simulink model "Neuron_Final"  (R2018a)
settings: Solver=VariableStepAuto  StartTime=0.0  StopTime=7200  RelTol=1e-3
settings Model: Creator=andys  LastModifiedBy=andys
settings CodeAppCC: StateflowObjectComments=on

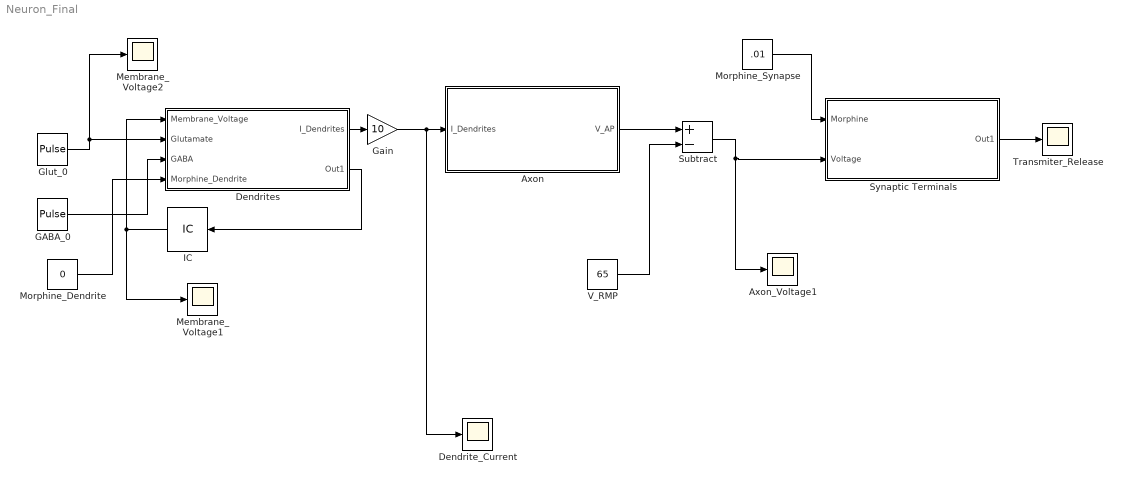
== system Neuron_Final ==
  Axon : Subsystem
  Axon_Voltage1 : Scope
  Dendrite_Current : Scope
  Dendrites : Subsystem
  GABA_0 : DiscretePulseGenerator  PulseType=Time based  Amplitude=0  Period=500  PulseWidth=0.1  PhaseDelay=500
  Gain : Gain  Gain=10
  Glut_0 : DiscretePulseGenerator  PulseType=Time based  Period=500  PulseWidth=0.1  PhaseDelay=500
  IC : InitialCondition  Value=-65
  Membrane_Voltage1 : Scope
  Membrane_Voltage2 : Scope
  Morphine_Dendrite : Constant  Value=0
  Morphine_Synapse : Constant  Value=.01
  Subtract : Sum  Inputs=+-
  Synaptic Terminals : Subsystem
  Transmiter_Release : Scope
  V_RMP : Constant  Value=65
  wires:
  Synaptic Terminals/1(Out1) -> Transmiter_Release/1
  Dendrites/1(I_Dendrites) -> Gain/1
  Glut_0/1 -> Dendrites/2(Glutamate), Membrane_Voltage2/1
  Dendrites/2(Out1) -> IC/1
  V_RMP/1 -> Subtract/2
  Subtract/1 -> Synaptic Terminals/2(Voltage), Axon_Voltage1/1
  IC/1 -> Dendrites/1(Membrane_Voltage), Membrane_Voltage1/1
  Axon/1(V_AP) -> Subtract/1
  Gain/1 -> Axon/1(I_Dendrites), Dendrite_Current/1
  Morphine_Dendrite/1 -> Dendrites/4(Morphine_Dendrite)
  Morphine_Synapse/1 -> Synaptic Terminals/1(Morphine)
  GABA_0/1 -> Dendrites/3(GABA)

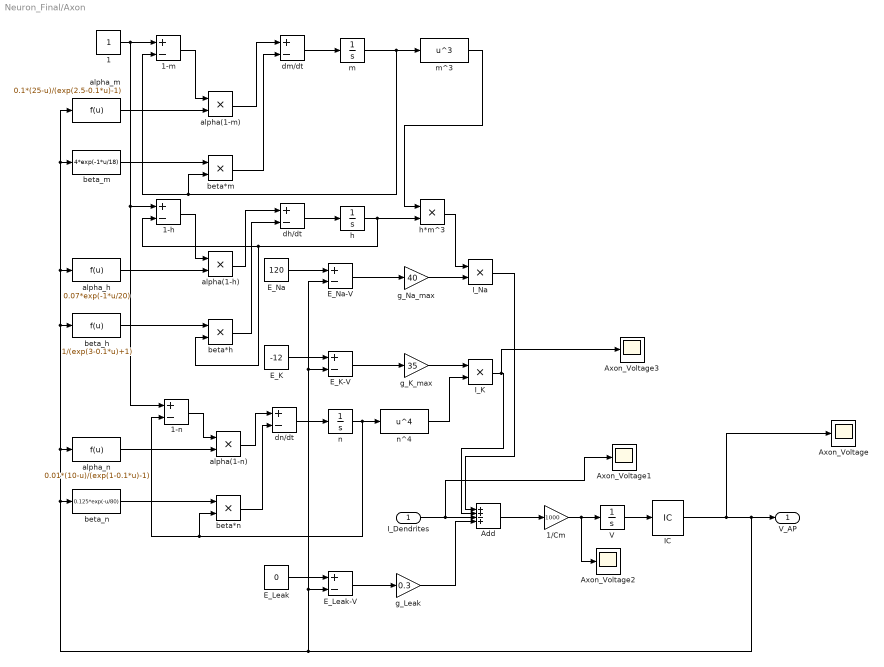
== system Neuron_Final/Axon ==
  I_Dendrites : Inport
  1 : Constant
  1-h : Sum  Inputs=+-
  1-m : Sum  Inputs=+-
  1-n : Sum  Inputs=+-
  1/Cm : Gain  Gain=1000
  Add : Sum  Inputs=++-+
  Axon_Voltage{,1..3} (4 alike) : Scope
  E_K : Constant  Value=-12
  E_K-V : Sum  Inputs=+-
  E_Leak : Constant  Value=0
  E_Leak-V : Sum  Inputs=+-
  E_Na : Constant  Value=120
  E_Na-V : Sum  Inputs=+-
  IC : InitialCondition  Value=0
  I_K : Product
  I_Na : Product
  V : Integrator
  alpha(1-h) : Product
  alpha(1-m) : Product
  alpha(1-n) : Product
  alpha_h : Fcn  Expr=0.07*exp(-1*u/20)
  alpha_m : Fcn  Expr=0.1*(25-u)/(exp(2.5-0.1*u)-1)
  alpha_n : Fcn  Expr=0.01*(10-u)/(exp(1-0.1*u)-1)
  beta*h : Product
  beta*m : Product
  beta*n : Product
  beta_h : Fcn  Expr=1/(exp(3-0.1*u)+1)
  beta_m : Fcn  Expr=4*exp(-1*u/18)
  beta_n : Fcn  Expr=0.125*exp(-u/80)
  dh/dt : Sum  Inputs=+-
  dm/dt : Sum  Inputs=+-
  dn/dt : Sum  Inputs=+-
  g_K_max : Gain  Gain=35
  g_Leak : Gain  Gain=0.3
  g_Na_max : Gain  Gain=40
  h : Integrator
  h*m^3 : Product
  m : Integrator
  m^3 : Fcn  Expr=u^3
  n : Integrator
  n^4 : Fcn  Expr=u^4
  V_AP : Outport
  wires:
  V/1 -> IC/1
  1/Cm/1 -> Axon_Voltage2/1, V/1
  E_Na/1 -> E_Na-V/1
  E_K/1 -> E_K-V/1
  E_Leak/1 -> E_Leak-V/1
  E_Leak-V/1 -> g_Leak/1
  E_K-V/1 -> g_K_max/1
  E_Na-V/1 -> g_Na_max/1
  Add/1 -> 1/Cm/1
  g_Leak/1 -> Add/4
  I_Dendrites/1 -> Axon_Voltage1/1, Add/3
  g_Na_max/1 -> I_Na/2
  g_K_max/1 -> I_K/1
  I_K/1 -> Axon_Voltage3/1, Add/2
  I_Na/1 -> Add/1
  IC/1 -> Axon_Voltage/1, alpha_m/1, beta_m/1, alpha_h/1, beta_h/1, alpha_n/1, beta_n/1, E_Na-V/2, E_K-V/2, E_Leak-V/2, V_AP/1
  n^4/1 -> I_K/2
  h*m^3/1 -> I_Na/1
  n/1 -> beta*n/2, 1-n/2, n^4/1
  m/1 -> m^3/1, beta*m/2, 1-m/2
  m^3/1 -> h*m^3/1
  h/1 -> 1-h/2, beta*h/2, h*m^3/2
  dn/dt/1 -> n/1
  dm/dt/1 -> m/1
  dh/dt/1 -> h/1
  1/1 -> 1-m/1, 1-h/1, 1-n/1
  alpha_m/1 -> alpha(1-m)/2
  1-m/1 -> alpha(1-m)/1
  alpha(1-m)/1 -> dm/dt/1
  beta_m/1 -> beta*m/1
  beta*m/1 -> dm/dt/2
  beta_h/1 -> beta*h/1
  alpha_h/1 -> alpha(1-h)/2
  1-h/1 -> alpha(1-h)/1
  alpha(1-h)/1 -> dh/dt/1
  beta*h/1 -> dh/dt/2
  1-n/1 -> alpha(1-n)/1
  alpha_n/1 -> alpha(1-n)/2
  alpha(1-n)/1 -> dn/dt/1
  beta_n/1 -> beta*n/1
  beta*n/1 -> dn/dt/2

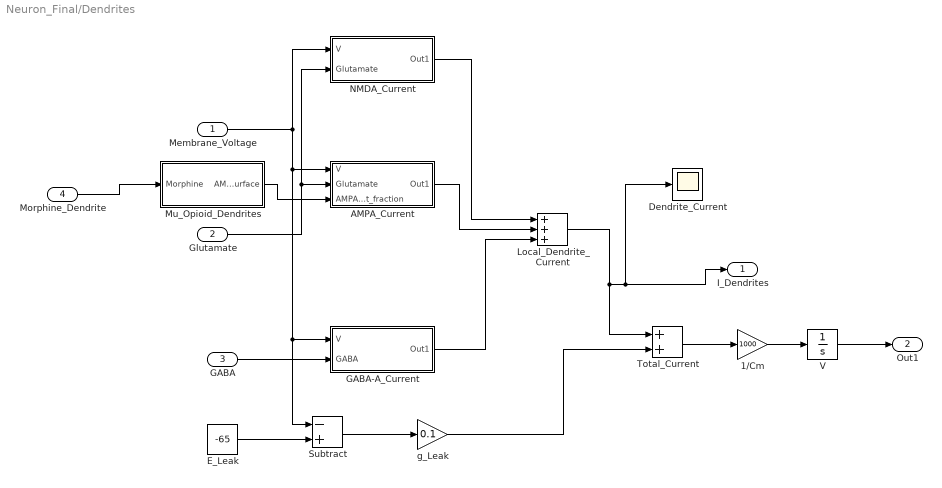
== system Neuron_Final/Dendrites ==
  Membrane_Voltage : Inport
  Glutamate : Inport  Port=2
  GABA : Inport  Port=3
  Morphine_Dendrite : Inport  Port=4
  1/Cm : Gain  Gain=1000
  AMPA_Current : Subsystem
  Dendrite_Current : Scope
  E_Leak : Constant  Value=-65
  GABA-A_Current : Subsystem
  Local_Dendrite_Current : Sum  Inputs=+++
  Mu_Opioid_Dendrites : Subsystem
  NMDA_Current : Subsystem
  Subtract : Sum  Inputs=-+
  Total_Current : Sum
  V : Integrator
  g_Leak : Gain  Gain=0.1
  I_Dendrites : Outport
  Out1 : Outport  Port=2
  wires:
  Membrane_Voltage/1 -> NMDA_Current/1(V), Subtract/1, GABA-A_Current/1(V), AMPA_Current/1(V)
  Glutamate/1 -> NMDA_Current/2(Glutamate), AMPA_Current/2(Glutamate)
  GABA/1 -> GABA-A_Current/2(GABA)
  AMPA_Current/1(Out1) -> Local_Dendrite_Current/2
  GABA-A_Current/1(Out1) -> Local_Dendrite_Current/3
  Local_Dendrite_Current/1 -> Dendrite_Current/1, I_Dendrites/1, Total_Current/1
  Total_Current/1 -> 1/Cm/1
  1/Cm/1 -> V/1
  V/1 -> Out1/1
  E_Leak/1 -> Subtract/2
  Subtract/1 -> g_Leak/1
  g_Leak/1 -> Total_Current/2
  NMDA_Current/1(Out1) -> Local_Dendrite_Current/1
  Morphine_Dendrite/1 -> Mu_Opioid_Dendrites/1("Morphine ")
  Mu_Opioid_Dendrites/1(AMPA_Surface) -> AMPA_Current/3(AMPA_current_fraction)

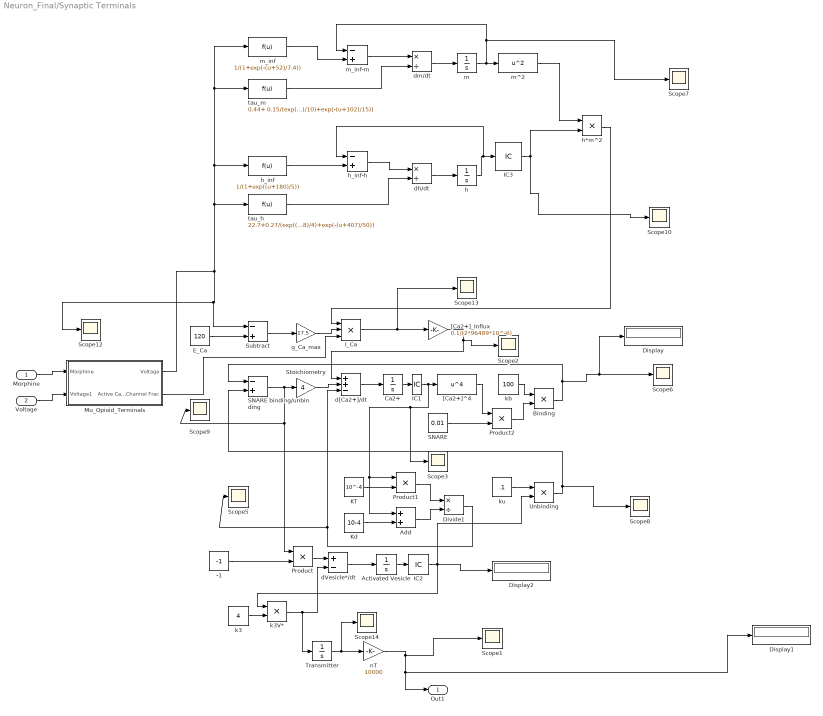
== system Neuron_Final/Synaptic Terminals ==
  Morphine : Inport
  Voltage : Inport  Port=2
  -1 : Constant  Value=-1
  Activated Vesicle : Integrator
  Add : Sum
  Binding : Product
  Ca2+ : Integrator
  Display : Display
  Display1 : Display
  Display2 : Display
  Divide1 : Product  Inputs=*/
  E_Ca : Constant  Value=120
  IC1 : InitialCondition  Value=0
  IC2 : InitialCondition  Value=0
  IC3 : InitialCondition
  I_Ca : Product  Inputs=3
  KT : Constant  Value=10^-4
  Kd : Constant  Value=10-4
  Mu_Opioid_Terminals : Subsystem
  Product : Product
  Product1 : Product
  Product2 : Product
  SNARE : Constant  Value=0.01
  SNARE binding/unbinding : Sum  Inputs=-+
  Scope{1..3,5..10,12..14} (12 alike) : Scope
  Stoichiometry : Gain  Gain=4
  Subtract : Sum  Inputs=-+
  Transmitter : Integrator
  Unbinding : Product
  "[Ca2+]^4" : Fcn  Expr=u^4
  "[Ca2+]_Influx" : Gain  Gain=0.1/(2*96489*10^-6)
  dVesicle*/dt : Sum  Inputs=+-
  d[Ca2+]/dt : Sum  Inputs=++-
  dh/dt : Product  Inputs=*/
  dm/dt : Product  Inputs=*/
  g_Ca_max : Gain  Gain=17.5
  h : Integrator
  h*m^2 : Product
  h_inf : Fcn  Expr=1/(1+exp((u+180)/5))
  h_inf-h : Sum  Inputs=-+
  k3 : Constant  Value=4
  k3V* : Product
  kb : Constant  Value=100
  ku : Constant  Value=.1
  m : Integrator
  m^2 : Fcn  Expr=u^2
  m_inf : Fcn  Expr=1/(1+exp(-(u+52)/7.4))
  m_inf-m : Sum  Inputs=-+
  nT : Gain  Gain=10000
  tau_h : Fcn  Expr=22.7+0.27/(exp((u+48)/4)+exp(-(u+407)/50))
  tau_m : Fcn  Expr=0.44+ 0.15/(exp((u+27)/10)+exp(-(u+102)/15))
  Out1 : Outport
  wires:
  d[Ca2+]/dt/1 -> Ca2+/1
  dVesicle*/dt/1 -> Activated Vesicle/1
  k3V*/1 -> Transmitter/1, dVesicle*/dt/2
  k3/1 -> k3V*/2
  Activated Vesicle/1 -> IC2/1
  Transmitter/1 -> Scope14/1, nT/1
  nT/1 -> Scope1/1, Display1/1, Out1/1
  kb/1 -> Binding/1
  E_Ca/1 -> Subtract/2
  Subtract/1 -> g_Ca_max/1
  g_Ca_max/1 -> I_Ca/2
  m/1 -> m_inf-m/1, Scope7/1, m^2/1
  m^2/1 -> h*m^2/1
  h*m^2/1 -> I_Ca/1
  I_Ca/1 -> Scope13/1, "[Ca2+]_Influx"/1
  "[Ca2+]_Influx"/1 -> Scope2/1, d[Ca2+]/dt/1
  SNARE binding/unbinding/1 -> Stoichiometry/1, Scope9/1, Product/1
  Stoichiometry/1 -> d[Ca2+]/dt/2
  Binding/1 -> Display/1, Scope6/1, SNARE binding/unbinding/1
  Unbinding/1 -> Scope8/1, SNARE binding/unbinding/2
  Ca2+/1 -> IC1/1
  IC1/1 -> Scope3/1, Add/1, Product1/1, "[Ca2+]^4"/1
  ku/1 -> Unbinding/1
  IC2/1 -> Display2/1, k3V*/1, Unbinding/2
  -1/1 -> Product/2
  Product/1 -> dVesicle*/dt/1
  Kd/1 -> Add/2
  KT/1 -> Product1/2
  Product1/1 -> Divide1/1
  Add/1 -> Divide1/2
  Divide1/1 -> Scope5/1, d[Ca2+]/dt/3
  h/1 -> h_inf-h/1, IC3/1
  m_inf/1 -> m_inf-m/2
  m_inf-m/1 -> dm/dt/1
  tau_m/1 -> dm/dt/2
  dm/dt/1 -> m/1
  dh/dt/1 -> h/1
  h_inf/1 -> h_inf-h/2
  h_inf-h/1 -> dh/dt/1
  tau_h/1 -> dh/dt/2
  IC3/1 -> Scope10/1, h*m^2/2
  "[Ca2+]^4"/1 -> Product2/1
  Product2/1 -> Binding/2
  SNARE/1 -> Product2/2
  Mu_Opioid_Terminals/1(Voltage) -> h_inf/1, tau_m/1, m_inf/1, tau_h/1, Subtract/1, Scope12/1
  Morphine/1 -> Mu_Opioid_Terminals/1(Morphine)
  Mu_Opioid_Terminals/2(Active Ca Channel Frac) -> I_Ca/3
  Voltage/1 -> Mu_Opioid_Terminals/2(Voltage1)

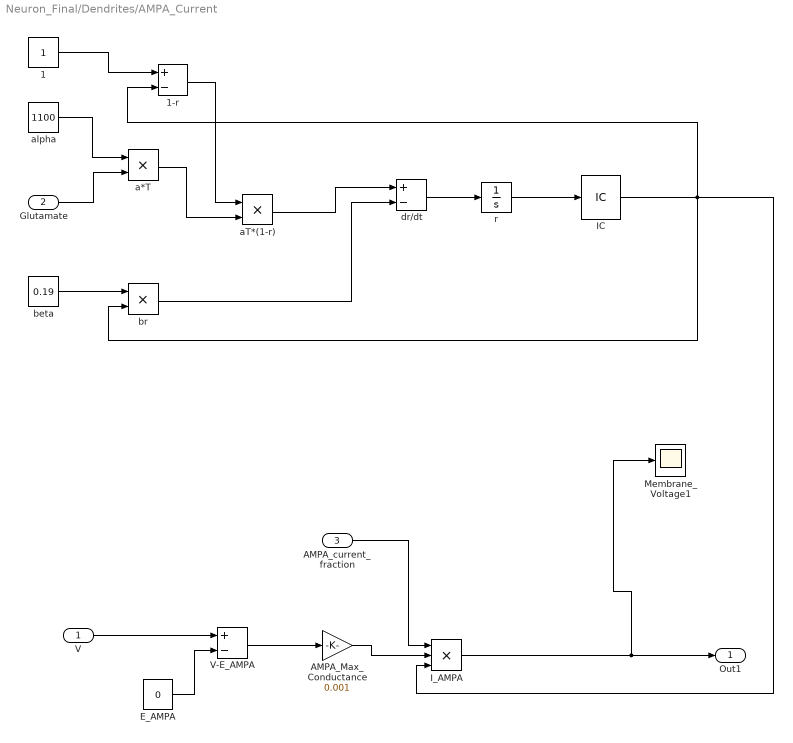
== system Neuron_Final/Dendrites/AMPA_Current ==
  V : Inport
  Glutamate : Inport  Port=2
  AMPA_current_fraction : Inport  Port=3
  1 : Constant
  1-r : Sum  Inputs=+-
  AMPA_Max_Conductance : Gain  Gain=0.001
  E_AMPA : Constant  Value=0
  IC : InitialCondition  Value=0
  I_AMPA : Product  Inputs=3
  Membrane_Voltage1 : Scope
  V-E_AMPA : Sum  Inputs=+-
  a*T : Product
  aT*(1-r) : Product
  alpha : Constant  Value=1100
  beta : Constant  Value=0.19
  br : Product
  dr/dt : Sum  Inputs=+-
  r : Integrator
  Out1 : Outport
  wires:
  E_AMPA/1 -> V-E_AMPA/2
  V-E_AMPA/1 -> AMPA_Max_Conductance/1
  V/1 -> V-E_AMPA/1
  I_AMPA/1 -> Membrane_Voltage1/1, Out1/1
  AMPA_Max_Conductance/1 -> I_AMPA/2
  dr/dt/1 -> r/1
  r/1 -> IC/1
  IC/1 -> I_AMPA/3, br/2, 1-r/2
  1/1 -> 1-r/1
  Glutamate/1 -> a*T/2
  alpha/1 -> a*T/1
  1-r/1 -> aT*(1-r)/1
  a*T/1 -> aT*(1-r)/2
  beta/1 -> br/1
  aT*(1-r)/1 -> dr/dt/1
  br/1 -> dr/dt/2
  AMPA_current_fraction/1 -> I_AMPA/1

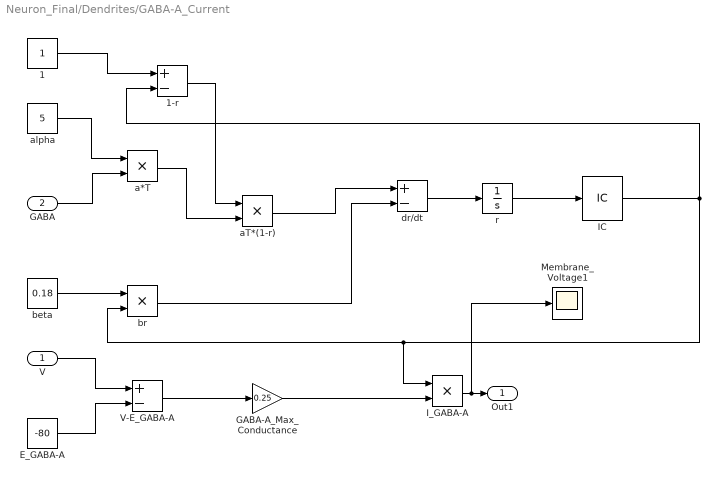
== system Neuron_Final/Dendrites/GABA-A_Current ==
  V : Inport
  GABA : Inport  Port=2
  1 : Constant
  1-r : Sum  Inputs=+-
  E_GABA-A : Constant  Value=-80
  GABA-A_Max_Conductance : Gain  Gain=0.25
  IC : InitialCondition  Value=0
  I_GABA-A : Product
  Membrane_Voltage1 : Scope
  V-E_GABA-A : Sum  Inputs=+-
  a*T : Product
  aT*(1-r) : Product
  alpha : Constant  Value=5
  beta : Constant  Value=0.18
  br : Product
  dr/dt : Sum  Inputs=+-
  r : Integrator
  Out1 : Outport
  wires:
  I_GABA-A/1 -> Membrane_Voltage1/1, Out1/1
  V/1 -> V-E_GABA-A/1
  E_GABA-A/1 -> V-E_GABA-A/2
  V-E_GABA-A/1 -> GABA-A_Max_Conductance/1
  GABA-A_Max_Conductance/1 -> I_GABA-A/2
  IC/1 -> br/2, I_GABA-A/1, 1-r/2
  dr/dt/1 -> r/1
  r/1 -> IC/1
  beta/1 -> br/1
  1/1 -> 1-r/1
  GABA/1 -> a*T/2
  1-r/1 -> aT*(1-r)/1
  alpha/1 -> a*T/1
  br/1 -> dr/dt/2
  a*T/1 -> aT*(1-r)/2
  aT*(1-r)/1 -> dr/dt/1

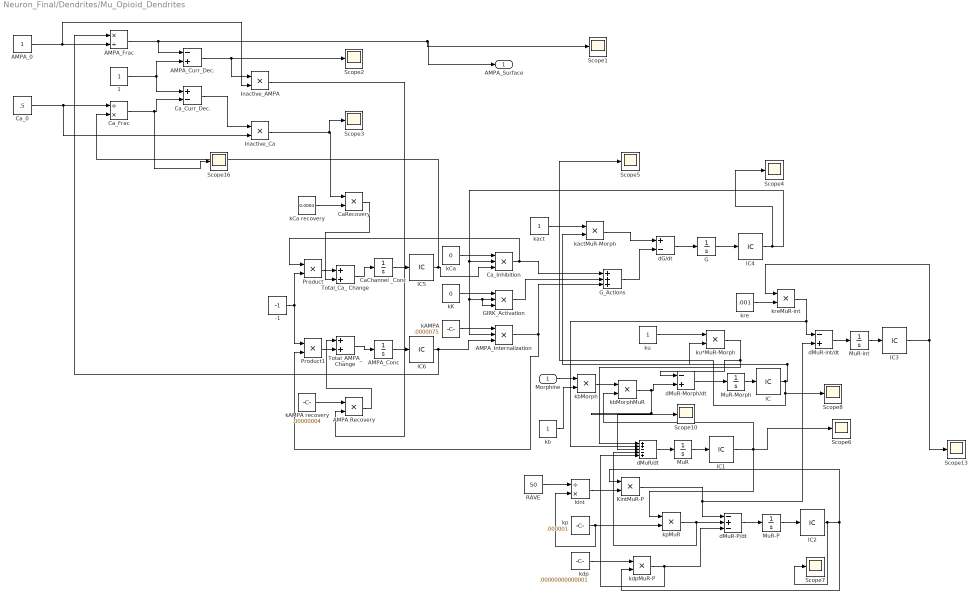
== system Neuron_Final/Dendrites/Mu_Opioid_Dendrites ==
  "Morphine " : Inport
  -1 : Constant  Value=-1
  1 : Constant
  AMPA Recovery : Product
  AMPA_0 : Constant
  AMPA_Conc : Integrator  InitialCondition=1
  AMPA_Curr_Dec. : Sum  Inputs=-+
  AMPA_Frac : Product  Inputs=*/
  AMPA_Internalization : Product  Inputs=3
  CaChannel _Conc : Integrator  InitialCondition=.5
  CaRecovery : Product
  Ca_0 : Constant  Value=.5
  Ca_Curr_Dec. : Sum  Inputs=+-
  Ca_Frac : Product  Inputs=/*
  Ca_Inhibition : Product  Inputs=3
  G : Integrator
  GIRK_Activation : Product  Inputs=3
  G_Actions : Sum  Inputs=+++
  IC{,2..4} (4 alike) : InitialCondition  Value=0
  IC1 : InitialCondition  Value=0.01
  IC5 : InitialCondition  Value=.5
  IC6 : InitialCondition
  Inactive_AMPA : Product
  Inactive_Ca : Product
  KintMuR-P : Product
  MuR : Integrator  InitialCondition=.01
  MuR-Morph : Integrator
  MuR-P : Integrator
  MuR-int : Integrator
  Product : Product
  Product1 : Product
  RAVE : Constant  Value=50
  Scope{1..8,10,13,16} (11 alike) : Scope
  Total_AMPA_ Change : Sum
  Total_Ca_ Change : Sum
  dG/dt : Sum  Inputs=+-
  dMuR-Morph/dt : Sum  Inputs=-+
  dMuR-P/dt : Sum  Inputs=-+-
  dMuR-int/dt : Sum  Inputs=-+
  dMuR/dt : Sum  Inputs=++--+
  kAMPA : Constant  Value=.0000075
  kAMPA recovery : Constant  Value=.00000004
  kCa : Constant  Value=0
  kCa recovery : Constant  Value=0.0004
  kK : Constant  Value=0
  kact : Constant
  kactMuR-Morph : Product
  kb : Constant
  kbMorph : Product
  kbMorphMuR : Product
  kdp : Constant  Value=.00000000000001
  kdpMuR-P : Product
  kint : Product  Inputs=/*
  kp : Constant  Value=.000001
  kpMuR : Product
  kre : Constant  Value=.001
  kreMuR-int : Product
  ku : Constant
  ku*MuR-Morph : Product
  AMPA_Surface : Outport
  wires:
  Ca_Inhibition/1 -> Product/1, G_Actions/1
  IC6/1 -> AMPA_Frac/1, AMPA_Internalization/3
  MuR-int/1 -> IC3/1
  AMPA_Curr_Dec./1 -> Scope2/1, Inactive_AMPA/1
  kactMuR-Morph/1 -> dG/dt/1
  kdp/1 -> kdpMuR-P/1
  dMuR/dt/1 -> MuR/1
  kre/1 -> kreMuR-int/2
  dG/dt/1 -> G/1
  Ca_Frac/1 -> Scope16/1, Ca_Curr_Dec./2
  Product1/1 -> Total_AMPA_ Change/2
  Product/1 -> Total_Ca_ Change/1
  kb/1 -> kbMorph/2
  AMPA Recovery/1 -> Total_AMPA_ Change/1
  Ca_Curr_Dec./1 -> Inactive_Ca/1
  Total_AMPA_ Change/1 -> AMPA_Conc/1
  Inactive_Ca/1 -> Scope3/1, CaRecovery/1
  Inactive_AMPA/1 -> AMPA Recovery/2
  kCa/1 -> Ca_Inhibition/1
  AMPA_Internalization/1 -> Product1/2, G_Actions/3
  CaRecovery/1 -> Total_Ca_ Change/2
  kdpMuR-P/1 -> dMuR/dt/5, dMuR-P/dt/3
  GIRK_Activation/1 -> G_Actions/2
  KintMuR-P/1 -> dMuR-int/dt/2, dMuR-P/dt/1
  kCa recovery/1 -> CaRecovery/2
  IC/1 -> Scope8/1, Scope5/1, kactMuR-Morph/2, ku*MuR-Morph/2
  AMPA_0/1 -> Inactive_AMPA/2, AMPA_Frac/2
  MuR/1 -> IC1/1
  IC4/1 -> Scope4/1, AMPA_Internalization/2, GIRK_Activation/3, GIRK_Activation/2, Ca_Inhibition/2
  kK/1 -> GIRK_Activation/1
  kbMorphMuR/1 -> Scope10/1, dMuR/dt/3, dMuR-Morph/dt/2
  MuR-P/1 -> IC2/1
  kp/1 -> kint/2, kpMuR/2
  dMuR-int/dt/1 -> MuR-int/1
  IC3/1 -> kreMuR-int/1, Scope13/1
  kAMPA/1 -> AMPA_Internalization/1
  G/1 -> IC4/1
  dMuR-Morph/dt/1 -> MuR-Morph/1
  kreMuR-int/1 -> dMuR/dt/2, dMuR-int/dt/1
  ku/1 -> ku*MuR-Morph/1
  ku*MuR-Morph/1 -> dMuR-Morph/dt/1, dMuR/dt/1
  kbMorph/1 -> kbMorphMuR/1
  kpMuR/1 -> dMuR/dt/4, dMuR-P/dt/2
  CaChannel _Conc/1 -> IC5/1
  MuR-Morph/1 -> IC/1
  IC5/1 -> Ca_Inhibition/3, Ca_Frac/2
  kAMPA recovery/1 -> AMPA Recovery/1
  1/1 -> AMPA_Curr_Dec./2, Ca_Curr_Dec./1
  kact/1 -> kactMuR-Morph/1
  AMPA_Conc/1 -> IC6/1
  "Morphine "/1 -> kbMorph/1
  -1/1 -> Product/2, Product1/1
  Ca_0/1 -> Inactive_Ca/2, Ca_Frac/1
  RAVE/1 -> kint/1
  IC1/1 -> Scope6/1, kpMuR/1, kbMorphMuR/2
  IC2/1 -> Scope7/1, kdpMuR-P/2, KintMuR-P/1
  AMPA_Frac/1 -> Scope1/1, AMPA_Surface/1, AMPA_Curr_Dec./1
  G_Actions/1 -> dG/dt/2
  dMuR-P/dt/1 -> MuR-P/1
  kint/1 -> KintMuR-P/2
  Total_Ca_ Change/1 -> CaChannel _Conc/1

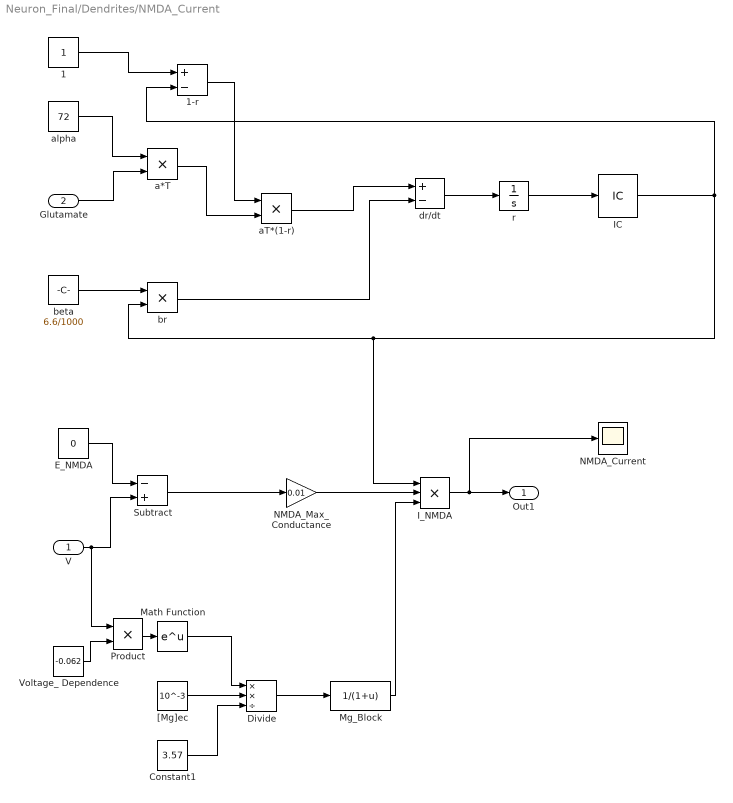
== system Neuron_Final/Dendrites/NMDA_Current ==
  V : Inport
  Glutamate : Inport  Port=2
  1 : Constant
  1-r : Sum  Inputs=+-
  Constant1 : Constant  Value=3.57
  Divide : Product  Inputs=**/
  E_NMDA : Constant  Value=0
  IC : InitialCondition  Value=0
  I_NMDA : Product  Inputs=3
  Math Function : Math  SaturateOnIntegerOverflow=on
  Mg_Block : Fcn  Expr=1/(1+u)
  NMDA_Current : Scope
  NMDA_Max_Conductance : Gain  Gain=0.01
  Product : Product
  Subtract : Sum  Inputs=-+
  Voltage_ Dependence : Constant  Value=-0.062
  "[Mg]ec" : Constant  Value=10^-3
  a*T : Product
  aT*(1-r) : Product
  alpha : Constant  Value=72
  beta : Constant  Value=6.6/1000
  br : Product
  dr/dt : Sum  Inputs=+-
  r : Integrator
  Out1 : Outport
  wires:
  NMDA_Max_Conductance/1 -> I_NMDA/2
  I_NMDA/1 -> NMDA_Current/1, Out1/1
  Voltage_ Dependence/1 -> Product/2
  "[Mg]ec"/1 -> Divide/2
  Product/1 -> Math Function/1
  Math Function/1 -> Divide/1
  Mg_Block/1 -> I_NMDA/3
  V/1 -> Product/1, Subtract/2
  Divide/1 -> Mg_Block/1
  Subtract/1 -> NMDA_Max_Conductance/1
  E_NMDA/1 -> Subtract/1
  Constant1/1 -> Divide/3
  r/1 -> IC/1
  1-r/1 -> aT*(1-r)/1
  1/1 -> 1-r/1
  Glutamate/1 -> a*T/2
  dr/dt/1 -> r/1
  aT*(1-r)/1 -> dr/dt/1
  alpha/1 -> a*T/1
  br/1 -> dr/dt/2
  a*T/1 -> aT*(1-r)/2
  IC/1 -> I_NMDA/1, br/2, 1-r/2
  beta/1 -> br/1

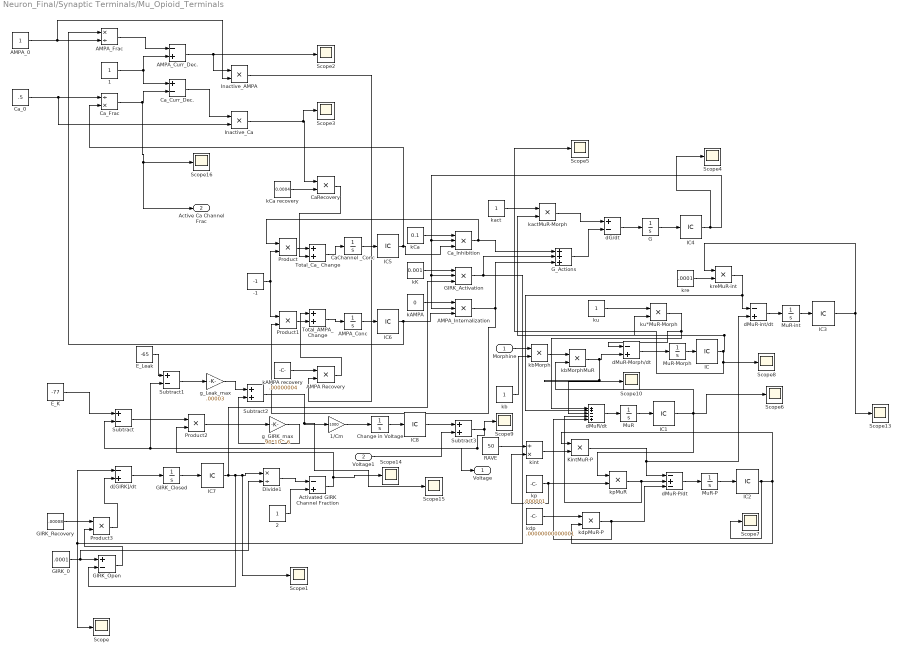
== system Neuron_Final/Synaptic Terminals/Mu_Opioid_Terminals ==
  Morphine : Inport
  Voltage1 : Inport  Port=2
  -1 : Constant  Value=-1
  1 : Constant
  1/Cm : Gain  Gain=1000
  2 : Constant
  AMPA Recovery : Product
  AMPA_0 : Constant
  AMPA_Conc : Integrator  InitialCondition=1
  AMPA_Curr_Dec. : Sum  Inputs=-+
  AMPA_Frac : Product  Inputs=*/
  AMPA_Internalization : Product  Inputs=3
  Activated GIRK Channel Fraction : Sum  Inputs=-+
  CaChannel _Conc : Integrator  InitialCondition=.5
  CaRecovery : Product
  Ca_0 : Constant  Value=.5
  Ca_Curr_Dec. : Sum  Inputs=+-
  Ca_Frac : Product  Inputs=/*
  Ca_Inhibition : Product  Inputs=3
  Change in Voltage : Integrator
  Divide1 : Product  Inputs=*/
  E_K : Constant  Value=-77
  E_Leak : Constant  Value=-65
  G : Integrator
  GIRK_0 : Constant  Value=.0001
  GIRK_Activation : Product  Inputs=3
  GIRK_Closed : Integrator  InitialCondition=.0001
  GIRK_Open : Sum  Inputs=+-
  GIRK_Recovery : Constant  Value=.00008
  G_Actions : Sum  Inputs=+++
  IC{,2..4,8} (5 alike) : InitialCondition  Value=0
  IC1 : InitialCondition  Value=0.01
  IC5 : InitialCondition  Value=.5
  IC6 : InitialCondition
  IC7 : InitialCondition  Value=.0001
  Inactive_AMPA : Product
  Inactive_Ca : Product
  KintMuR-P : Product
  MuR : Integrator  InitialCondition=.01
  MuR-Morph : Integrator
  MuR-P : Integrator
  MuR-int : Integrator
  Product{,1..3} (4 alike) : Product
  RAVE : Constant  Value=50
  Scope{,1..10,13..16} (15 alike) : Scope
  Subtract : Sum  Inputs=+-
  Subtract1 : Sum  Inputs=+-
  Subtract2 : Sum
  Subtract3 : Sum
  Total_AMPA_ Change : Sum
  Total_Ca_ Change : Sum
  dG/dt : Sum  Inputs=+-
  dMuR-Morph/dt : Sum  Inputs=-+
  dMuR-P/dt : Sum  Inputs=-+-
  dMuR-int/dt : Sum  Inputs=-+
  dMuR/dt : Sum  Inputs=++--+
  d[GIRK]/dt : Sum  Inputs=-+
  g_GIRK_max : Gain  Gain=90*10^-6
  g_Leak_max : Gain  Gain=.00003
  kAMPA : Constant  Value=0
  kAMPA recovery : Constant  Value=.00000004
  kCa : Constant  Value=0.1
  kCa recovery : Constant  Value=0.0004
  kK : Constant  Value=0.001
  kact : Constant
  kactMuR-Morph : Product
  kb : Constant
  kbMorph : Product
  kbMorphMuR : Product
  kdp : Constant  Value=.00000000000001
  kdpMuR-P : Product
  kint : Product  Inputs=/*
  kp : Constant  Value=.000001
  kpMuR : Product
  kre : Constant  Value=.0001
  kreMuR-int : Product
  ku : Constant
  ku*MuR-Morph : Product
  Voltage : Outport
  Active Ca Channel Frac : Outport  Port=2
  wires:
  g_GIRK_max/1 -> Subtract2/2
  g_Leak_max/1 -> Subtract2/1
  Change in Voltage/1 -> IC8/1
  Subtract1/1 -> g_Leak_max/1
  Ca_Inhibition/1 -> Product/1, G_Actions/1
  IC6/1 -> AMPA_Frac/1, AMPA_Internalization/3
  MuR-int/1 -> IC3/1
  AMPA_Curr_Dec./1 -> Scope2/1, Inactive_AMPA/1
  kactMuR-Morph/1 -> dG/dt/1
  kdp/1 -> kdpMuR-P/1
  dMuR/dt/1 -> MuR/1
  kre/1 -> kreMuR-int/2
  dG/dt/1 -> G/1
  Ca_Frac/1 -> Active Ca Channel Frac/1, Scope16/1, Ca_Curr_Dec./2
  Product1/1 -> Total_AMPA_ Change/2
  Product/1 -> Total_Ca_ Change/1
  kb/1 -> kbMorph/2
  AMPA Recovery/1 -> Total_AMPA_ Change/1
  Ca_Curr_Dec./1 -> Inactive_Ca/1
  Total_AMPA_ Change/1 -> AMPA_Conc/1
  Inactive_Ca/1 -> Scope3/1, CaRecovery/1
  Inactive_AMPA/1 -> AMPA Recovery/2
  kCa/1 -> Ca_Inhibition/1
  AMPA_Internalization/1 -> Product1/2, G_Actions/3
  CaRecovery/1 -> Total_Ca_ Change/2
  kdpMuR-P/1 -> dMuR/dt/5, dMuR-P/dt/3
  GIRK_Activation/1 -> d[GIRK]/dt/1, Scope/1, G_Actions/2
  KintMuR-P/1 -> dMuR-int/dt/2, dMuR-P/dt/1
  kCa recovery/1 -> CaRecovery/2
  IC/1 -> Scope8/1, Scope5/1, kactMuR-Morph/2, ku*MuR-Morph/2
  AMPA_0/1 -> Inactive_AMPA/2, AMPA_Frac/2
  MuR/1 -> IC1/1
  IC4/1 -> Scope4/1, AMPA_Internalization/2, GIRK_Activation/2, Ca_Inhibition/2
  kK/1 -> GIRK_Activation/1
  kbMorphMuR/1 -> Scope10/1, dMuR/dt/3, dMuR-Morph/dt/2
  MuR-P/1 -> IC2/1
  kp/1 -> kint/2, kpMuR/2
  dMuR-int/dt/1 -> MuR-int/1
  IC3/1 -> kreMuR-int/1, Scope13/1
  kAMPA/1 -> AMPA_Internalization/1
  G/1 -> IC4/1
  dMuR-Morph/dt/1 -> MuR-Morph/1
  kreMuR-int/1 -> dMuR/dt/2, dMuR-int/dt/1
  ku/1 -> ku*MuR-Morph/1
  E_Leak/1 -> Subtract1/1
  ku*MuR-Morph/1 -> dMuR-Morph/dt/1, dMuR/dt/1
  GIRK_Closed/1 -> IC7/1
  1/Cm/1 -> Change in Voltage/1
  kbMorph/1 -> kbMorphMuR/1
  Divide1/1 -> Activated GIRK Channel Fraction/1
  E_K/1 -> Subtract/1
  Product2/1 -> g_GIRK_max/1
  IC7/1 -> GIRK_Activation/3, GIRK_Open/2, Scope1/1, Divide1/1
  kpMuR/1 -> dMuR/dt/4, dMuR-P/dt/2
  CaChannel _Conc/1 -> IC5/1
  GIRK_0/1 -> Divide1/2, GIRK_Open/1
  MuR-Morph/1 -> IC/1
  IC5/1 -> Ca_Inhibition/3, Ca_Frac/2
  GIRK_Recovery/1 -> Product3/1
  Subtract/1 -> Product2/1
  Activated GIRK Channel Fraction/1 -> Scope14/1, Product2/2
  kAMPA recovery/1 -> AMPA Recovery/1
  Product3/1 -> d[GIRK]/dt/2
  1/1 -> AMPA_Curr_Dec./2, Ca_Curr_Dec./1
  d[GIRK]/dt/1 -> GIRK_Closed/1
  kact/1 -> kactMuR-Morph/1
  AMPA_Conc/1 -> IC6/1
  Morphine/1 -> kbMorph/1
  -1/1 -> Product/2, Product1/1
  Ca_0/1 -> Inactive_Ca/2, Ca_Frac/1
  RAVE/1 -> kint/1
  IC1/1 -> Scope6/1, kpMuR/1, kbMorphMuR/2
  IC2/1 -> Scope7/1, kdpMuR-P/2, KintMuR-P/1
  AMPA_Frac/1 -> AMPA_Curr_Dec./1
  G_Actions/1 -> dG/dt/2
  dMuR-P/dt/1 -> MuR-P/1
  2/1 -> Activated GIRK Channel Fraction/2
  GIRK_Open/1 -> Product3/2
  Subtract2/1 -> Scope15/1, 1/Cm/1
  kint/1 -> KintMuR-P/2
  Total_Ca_ Change/1 -> CaChannel _Conc/1
  IC8/1 -> Subtract3/1
  Voltage1/1 -> Subtract3/2
  Subtract3/1 -> Scope9/1, Voltage/1, Subtract1/2, Subtract/2
